simulink model "Case1"  (R2022b)
settings: Solver=FixedStepAuto  StartTime=0.0  StopTime=20  FixedStep=1e-6  RelTol=1e-3
libraries: spsSeriesRLCBranchLib x5, spsCurrentMeasurementLib x3, spsVoltageMeasurementLib x2, spsDCMachineLib x1, spsPWMGeneratorDCDCLib x1, spsMosfetLib x1, spsDiodeLib x1, spsDCVoltageSourceLib x1, spspowerguiLib x1
settings Model: Creator=enes_  LastModifiedBy=AhmetAkman
settings DebuggingCC: UnconnectedInputMsg=warning  UnconnectedOutputMsg=warning  UnconnectedLineMsg=warning
settings ModelReferenceCC: EnableRefExpFcnMdlSchedulingChecks=on
settings RTWCC: DLArmComputeVersion=19.05

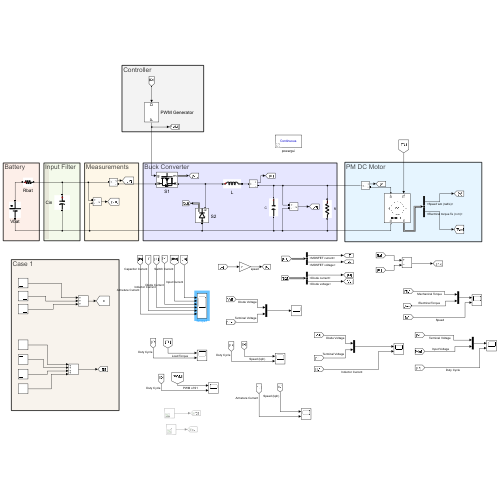
[thumbnail: Simulink's stored preview of the top-level diagram]
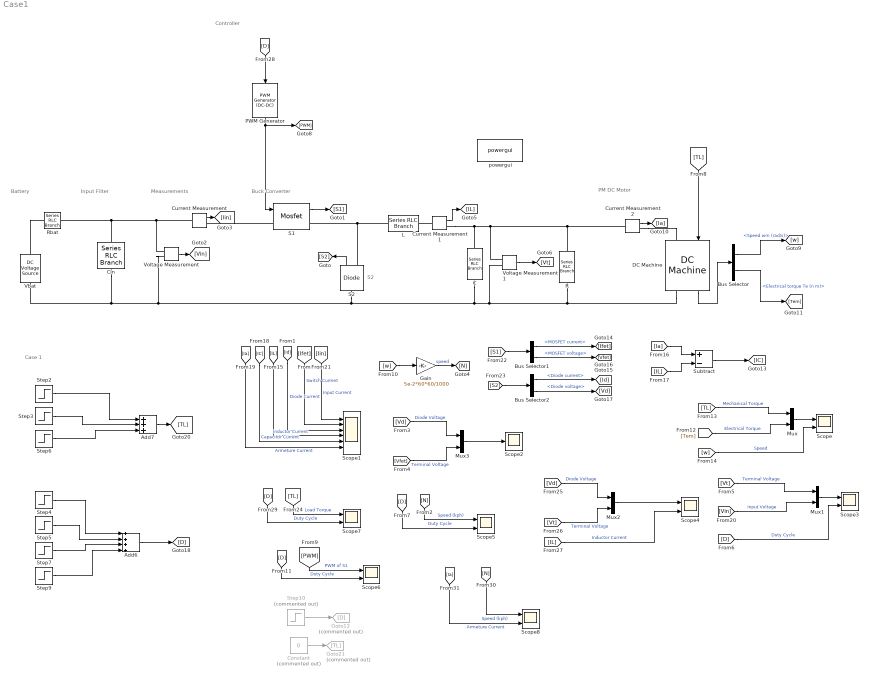
== system Case1 ==
  note: S2
  note: Battery
  note: Input Filter
  note: Measurements
  note: Buck Converter
  note: Controller
  note: PM DC Motor
  note: Case 1
  Add6 : Sum  Inputs=++++
  Add7 : Sum  Inputs=+++
  Bus Selector : BusSelector  OutputSignals=Speed wm (rad/s),Electrical torque Te (n m)
  Bus Selector1 : BusSelector  OutputSignals=MOSFET current,MOSFET voltage
  Bus Selector2 : BusSelector  OutputSignals=Diode current,Diode voltage
  C : spsSeriesRLCBranchLib/Series RLC Branch  LConnTagsString=__new0  RConnTagsString=__new0  BranchType=C  Resistance=1e-5  Inductance=1e-3  SetiL0=off  InitialCurrent=0  Capacitance=100e-6  Setx0=off  InitialVoltage=0  Measurements=None
  Cin : spsSeriesRLCBranchLib/Series RLC Branch  LConnTagsString=__new0  RConnTagsString=__new0  BranchType=C  Resistance=0.2  Inductance=1e-3  SetiL0=off  InitialCurrent=0  Capacitance=100e-6  Setx0=off  InitialVoltage=0  Measurements=None
  Constant : Constant  Commented=on  Value=0
  Current Measurement : spsCurrentMeasurementLib/Current Measurement  PhasorSimulation=off  OutputType=Complex  PSBequivalent=0
  Current Measurement1 : spsCurrentMeasurementLib/Current Measurement  PhasorSimulation=off  OutputType=Complex  PSBequivalent=0
  Current Measurement2 : spsCurrentMeasurementLib/Current Measurement  PhasorSimulation=off  OutputType=Complex  PSBequivalent=0
  DC Machine : spsDCMachineLib/DC Machine  PresetModel=No  MechanicalLoad=Torque TL  FieldType=Permanent magnet  ShowDetailedParameters=on  MeasurementBus=off  RLa=[0.0738 0.00012]  RLf="[ 240  120]"  Laf=1.8  MachineConstant=Torque constant (N.m/A)  Ke=1.8  Kt=0.3416  J=0.0130  Bm=0.002076  Tf=0.2  w0=0  Ifinit=1  TsPowergui=0  TsBlock=-1
  Gain : Gain  Gain=5e-2*60*60/1000
  Goto12 : Goto  Commented=on  GotoTag=D
  Goto21 : Goto  Commented=on  GotoTag=TL
  L : spsSeriesRLCBranchLib/Series RLC Branch  LConnTagsString=__new0  RConnTagsString=__new0  BranchType=L  Resistance=1e-3  Inductance=400e-6  SetiL0=off  InitialCurrent=0  Capacitance=1e-6  Setx0=off  InitialVoltage=0  Measurements=None
  Mux{,1..3} (4 alike) : Mux  Inputs=2
  PWM Generator : spsPWMGeneratorDCDCLib/PWM Generator (DC-DC)  Fsw=20e3  Ts=0
  R : spsSeriesRLCBranchLib/Series RLC Branch  LConnTagsString=__new0  RConnTagsString=__new0  BranchType=R  Resistance=100  Inductance=1e-3  SetiL0=off  InitialCurrent=0  Capacitance=100e-6  Setx0=off  InitialVoltage=0  Measurements=None
  Rbat : spsSeriesRLCBranchLib/Series RLC Branch  LConnTagsString=__new0  RConnTagsString=__new0  BranchType=R  Resistance=0.2  Inductance=1e-3  SetiL0=off  InitialCurrent=0  Capacitance=1e-6  Setx0=off  InitialVoltage=0  Measurements=None
  S1 : spsMosfetLib/Mosfet  Ron=1e-3  Lon=0  Rd=1e-3  Vfd=0  IC=0  Rs=inf  Cs=inf  Measurements=on
  S2 : spsDiodeLib/Diode  Ron=1e-3  Lon=0  Vf=0  IC=0  UseSnubber=off  Rs=inf  Cs=inf  Measurements=on
  Scope{,3..8} (7 alike) : Scope  NumInputPorts=2
  Scope1 : Scope  NumInputPorts=6
  Scope2 : Scope
  Step10 : Step  Commented=on  After=0.92  SampleTime=0
  Step2 : Step  Time=3  After=1.75  SampleTime=0
  Step3 : Step  Time=6  After=-1  SampleTime=0
  Step4 : Step  After=0.8  SampleTime=0
  Step5 : Step  Time=4  After=-0.3  SampleTime=0
  Step6 : Step  Time=12  After=-0.75  SampleTime=0
  Step7 : Step  Time=10  After=0.4  SampleTime=0
  Step9 : Step  Time=14  After=-0.9  SampleTime=0
  Subtract : Sum  Inputs=+-
  Vbat : spsDCVoltageSourceLib/DC Voltage Source  Amplitude=52  Measurements=None
  Voltage Measurement : spsVoltageMeasurementLib/Voltage Measurement  PhasorSimulation=off  OutputType=Complex  PSBequivalent=0
  Voltage Measurement1 : spsVoltageMeasurementLib/Voltage Measurement  PhasorSimulation=off  OutputType=Complex  PSBequivalent=0
  powergui : spspowerguiLib/powergui  Priority=1  SimulationMode=Continuous  SampleTime=50e-6  frequency=60  Iterations=50  frequencyindice=0  Pbase=100e6  ErrMax=1e-4  UnitsV=kV  UnitsW=MW  buscounter=0  FunctionMessages=off  echomessages=off  EnableUseOfTLC=off  CurrentSourceSwitches=off  DisableSnubberDevices=off  DisableRonSwitches=off  DisableVfSwitches=off  DisplayEquations=off  AutomaticDiscreteSolvers=off  SolverType=Tustin/Backward Euler (TBE)  Interpol=off  ExternalGateDelay=off  methode=off  Ts=100  x0status=blocks  SPID=on  SwTol=0  HookPort=off  NonlinearTolerance=1e-4  nMaxIteration=100  ContinueOnMaxIteration=off  RestoreLinks=warning  ResistiveCurrentMeasurement=off  Frange=[0:2:500]  Ylog=off  Xlog=on  ShowGrid=off  save=off  variable=ZData  structure=0  ZoomFFT=off  StartTime=0.0  cycles=1  DisplayStyle=1  fundamental=60  FreqAxis=off  MaxFrequency=1000  frequencyindicesteady=1  RmsSteady=1  display=off
  wires:
  DC Machine/1 -> Bus Selector/1
  Bus Selector/1 -> [w]  "<Speed wm (rad/s)>"
  Bus Selector/2 -> [Tem]  "<Electrical torque Te (n m)>"
  Voltage Measurement/1 -> [Vin]
  Current Measurement/1 -> [Iin]
  Gain/1 -> [N]  "speed"
  Voltage Measurement1/1 -> [Vt]
  Current Measurement1/1 -> [IL]
  PWM Generator/1 -> S1/1, [PWM]
  S1/1 -> [S1]
  S2/1 -> [S2]
  Current Measurement2/1 -> [Ia]
  [w] -> Gain/1
  [TL] -> Mux/1  "Mechanical Torque"
  [Tem] -> Mux/2  "Electrical Torque"
  Mux/1 -> Scope/1
  [w] -> Scope/2  "Speed"
  [Ia] -> Subtract/1
  [IL] -> Scope1/4  "Inductor Current"
  [IL] -> Subtract/2
  Subtract/1 -> [IC]
  [IC] -> Scope1/5  "Capacitor Current"
  [Ia] -> Scope1/6  "Armeture Current"
  [Iin] -> Scope1/1  "Input Current"
  [D] -> Scope3/2  "Duty Cycle"
  [Vt] -> Mux1/1  "Terminal Voltage"
  [Vin] -> Mux1/2  "Input Voltage"
  Mux1/1 -> Scope3/1
  [S1] -> Bus Selector1/1
  Bus Selector1/1 -> [Ifet]  "<MOSFET current>"
  [S2] -> Bus Selector2/1
  Bus Selector2/1 -> [Id]  "<Diode current>"
  Bus Selector1/2 -> [Vfet]  "<MOSFET voltage>"
  Bus Selector2/2 -> [Vd]  "<Diode voltage>"
  [Vt] -> Mux2/2  "Terminal Voltage"
  [Vd] -> Mux2/1  "Diode Voltage"
  Mux2/1 -> Scope4/1
  [IL] -> Scope4/2  "Inductor Current"
  [Ifet] -> Scope1/2  "Switch Current"
  [Id] -> Scope1/3  "Diode Current"
  [D] -> PWM Generator/1
  Add7/1 -> [TL]
  Step3/1 -> Add7/2
  Step2/1 -> Add7/1
  Step4/1 -> Add6/1
  Add6/1 -> [D]
  Step5/1 -> Add6/2
  Step7/1 -> Add6/3
  [TL] -> DC Machine/1
  [Vfet] -> Mux3/2  "Terminal Voltage"
  Mux3/1 -> Scope2/1
  [Vd] -> Mux3/1  "Diode Voltage"
  [N] -> Scope5/1  "Speed (kph)"
  [D] -> Scope5/2  "Duty Cycle"
  [PWM] -> Scope6/1  "PWM of S1"
  [D] -> Scope6/2  "Duty Cycle"
  [D] -> Scope7/2  "Duty Cycle"
  [TL] -> Scope7/1  "Load Torque"
  Step9/1 -> Add6/4
  Step10/1 -> Goto12/1
  Constant/1 -> Goto21/1
  [N] -> Scope8/1  "Speed (kph)"
  [Ia] -> Scope8/2  "Armeture Current"
  Step6/1 -> Add7/3
  connections:
  Voltage Measurement1/LConn1 -- Current Measurement2/LConn1 -- R/LConn1 -- Current Measurement1/RConn1 -- C/LConn1
  Current Measurement1/LConn1 -- L/RConn1
  Current Measurement2/RConn1 -- DC Machine/LConn1
  S2/RConn1 -- L/LConn1 -- S1/RConn1
  S1/LConn1 -- Current Measurement/RConn1
  Voltage Measurement/LConn2 -- Vbat/LConn1 -- Cin/RConn1 -- S2/LConn1 -- DC Machine/RConn1 -- R/RConn1 -- Voltage Measurement1/LConn2 -- C/RConn1
  Rbat/LConn1 -- Vbat/RConn1
  Voltage Measurement/LConn1 -- Rbat/RConn1 -- Cin/LConn1 -- Current Measurement/LConn1
